simulink library "roombaCtrl"  (R2017b)
settings: Solver=VariableStepAuto  StartTime=0.0  StopTime=10.0  RelTol=1e-3
settings Model: Creator=Hoa  LastModifiedBy=Hoa

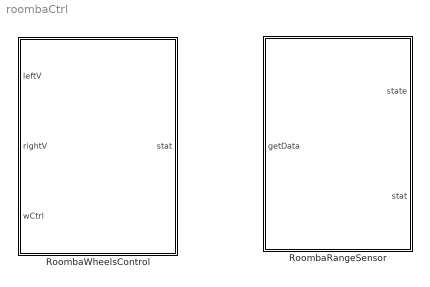
== system roombaCtrl ==
  RoombaRangeSensor : Subsystem
  RoombaWheelsControl : Subsystem

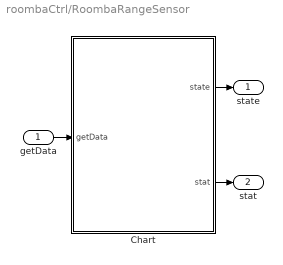
== system roombaCtrl/RoombaRangeSensor ==
  getData : Inport
  Chart : Stateflow chart  TreatAsAtomicUnit=on
  state : Outport
  stat : Outport  Port=2
  wires:
  Chart/2(stat) -> stat/1
  Chart/1(state) -> state/1
  getData/1 -> Chart/1(getData)

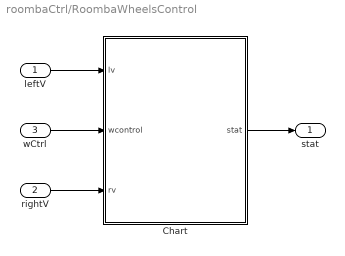
== system roombaCtrl/RoombaWheelsControl ==
  leftV : Inport
  rightV : Inport  Port=2
  wCtrl : Inport  Port=3
  Chart : Stateflow chart  TreatAsAtomicUnit=on
  stat : Outport
  wires:
  rightV/1 -> Chart/3(rv)
  leftV/1 -> Chart/1(lv)
  wCtrl/1 -> Chart/2(wcontrol)
  Chart/1(stat) -> stat/1

== stateflow chart roombaCtrl/RoombaRangeSensor/Chart ==
  state NO_OP
    en:
    data = [0;0;0;0;0;0]
    stat = 0;
  state RESET
    en:
    state = data
  state START
    en:
    coder.extrinsic('RangeStateRoomba')
    data = RangeStateRoomba(so)
    stat = 1;
  (default) -> NO_OP : {
      | 	coder.extrinsic('RoombaWiFiInit')
      | 	so = RoombaWiFiInit('10.0.0.1','full')
      | }
  RESET -> NO_OP : [getData==0]
  NO_OP -> START : [getData==1]
  START -> RESET : after(0.5,sec)
  data: state output double size=6; stat output; so local; getData input; data local

== stateflow chart roombaCtrl/RoombaWheelsControl/Chart ==
  state NO_OP
    en:
    stat = 0;
  state STOP
    en:
    SetWheelVelRoomba(so,0,0)
  state START
    en:
    coder.extrinsic('SetWheelVelRoomba')
    SetWheelVelRoomba(so,rv,lv)
    stat = 1;
  (default) -> NO_OP : {
      | 	coder.extrinsic('RoombaWiFiInit')
      | 	so = RoombaWiFiInit('10.0.0.1','full')
      | }
  STOP -> NO_OP : after(0.5,sec)
  NO_OP -> START : [wcontrol==1]
  START -> STOP : [wcontrol==0]
  data: so local; lv input; wcontrol input; rv input; stat output
